simulink model "mckblock"  (Simulink 6.6)
settings: Solver=ode45  StartTime=0.0  StopTime=10.0  MaxStep=.001  RelTol=1e-3
InitFcn:
  | mck
undefined symbols (not defined in the file): c, k, m, v0
settings Model: Creator=w006jcs  LastModifiedBy=w006jcs  ExtModeAutoUpdateStatusClock=off

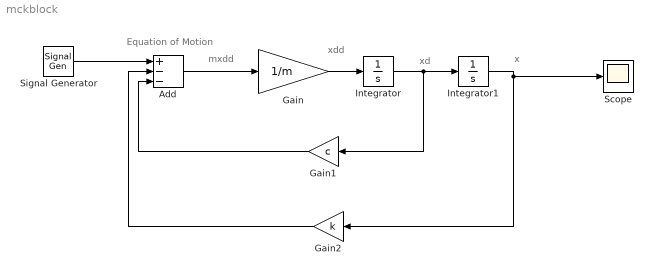
== system mckblock ==
  note: xdd
  note: xd
  note: x
  note: mxdd
  note: Equation of Motion
  Add : Sum  Inputs=+--  OutScaling=2^-10
  Gain : Gain  Gain=1/m
  Gain1 : Gain  Orientation=left  Gain=c
  Gain2 : Gain  Orientation=left  Gain=k
  Integrator : Integrator  InitialCondition=v0
  Integrator1 : Integrator
  Scope : Scope
  Signal Generator : SignalGenerator
  wires:
  Signal Generator/1 -> Add/1
  Add/1 -> Gain/1
  Gain/1 -> Integrator/1
  Integrator/1 -> Integrator1/1, Gain1/1
  Integrator1/1 -> Gain2/1, Scope/1
  Gain2/1 -> Add/2
  Gain1/1 -> Add/3
